simulink model "lateralControlTests"  (R2022a)
settings: Solver=VariableStepAuto  StartTime=0  StopTime=20  FixedStep=0.01  RelTol=1e-3
values from neighbouring files (symbols this model uses):
  Klat = place(A, B, poles)    [lat_sim_parameters.m]    (also in tuneLateralController.m)
  lr = 1.6    [acc_sim_parameters.m]    (also in lat_sim_parameters.m = 2; tuneLateralController.m = 2)
  m = 1575    [acc_sim_parameters.m]    (also in lat_sim_parameters.m = 2000; tuneLateralController.m = 2000)
  vx0 = 20    [lat_sim_parameters.m]    (also in tuneLateralController.m)
libraries: autolibshared x1
settings Model: Creator=Fernando VM  LastModifiedBy=fvall
settings SolverCC: AlgebraicLoopSolver=TrustRegion
settings DataIOCC: ExternalInput=[dt, da, dd]  ReturnWorkspaceOutputs=off
settings DebuggingCC: UnconnectedInputMsg=warning  UnconnectedOutputMsg=warning  UnconnectedLineMsg=warning  SFMachineParentedDataDiag=warning  ArithmeticOperatorsInVariantConditions=warning
settings SFSimCC: CustomCodeUndefinedFunction=UseInterfaceOnly

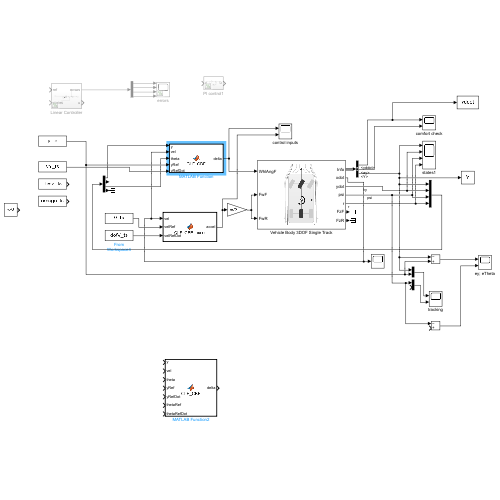
[thumbnail: Simulink's stored preview of the top-level diagram]
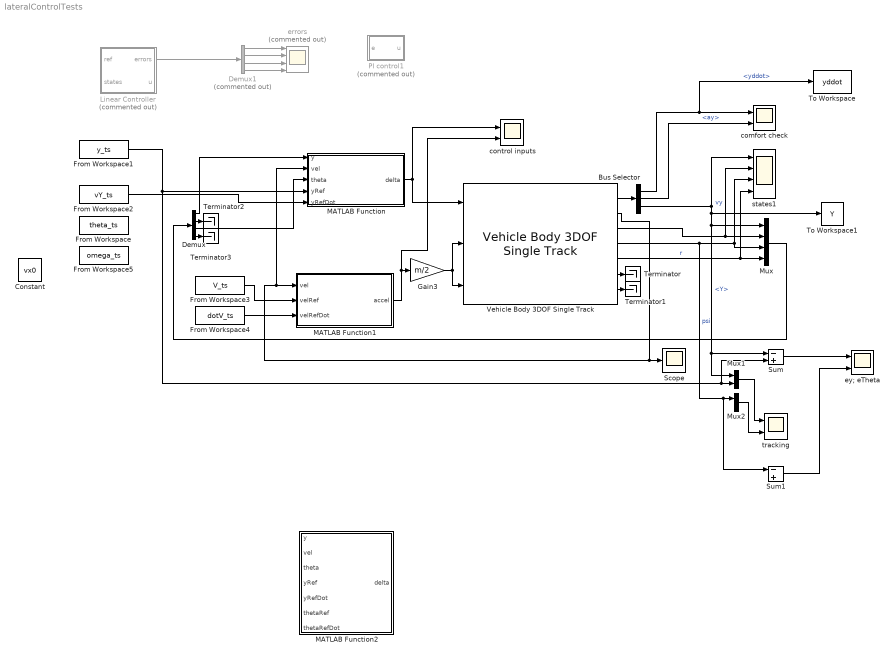
== system lateralControlTests ==
  Bus Selector : BusSelector  OutputSignals=BdyFrm.Cg.Acc.yddot,BdyFrm.Cg.Acc.ay,InertFrm.Cg.Disp.Y
  Constant : Constant  Value=vx0
  Demux : Demux
  Demux1 : Demux  Commented=on
  From Workspace : FromWorkspace  VariableName=theta_ts
  From Workspace1 : FromWorkspace  VariableName=y_ts
  From Workspace2 : FromWorkspace  VariableName=vY_ts
  From Workspace3 : FromWorkspace  VariableName=V_ts
  From Workspace4 : FromWorkspace  VariableName=dotV_ts
  From Workspace5 : FromWorkspace  VariableName=omega_ts
  Gain3 : Gain  Gain=m/2
  Linear Controller : Subsystem  Commented=on
  MATLAB Function : MATLAB Function  TreatAsAtomicUnit=on
  MATLAB Function1 : MATLAB Function  TreatAsAtomicUnit=on
  MATLAB Function2 : MATLAB Function  TreatAsAtomicUnit=on
  Mux : Mux
  Mux1 : Mux  Inputs=2
  Mux2 : Mux  Inputs=2
  PI control1 : Subsystem  Commented=on
  Scope : Scope
  Sum : Sum  Inputs=-+
  Sum1 : Sum  Inputs=-+
  Terminator{,1..3} (4 alike) : Terminator
  To Workspace : ToWorkspace  VariableName=yddot  SaveFormat=Timeseries  SampleTime=-1
  To Workspace1 : ToWorkspace  VariableName=Y  SaveFormat=Timeseries  SampleTime=-1
  Vehicle Body 3DOF Single Track : autolibshared/Vehicle Body 3DOF Single Track  trackMode=Single (bicycle)  inputMode=External longitudinal forces  frontSteerMode=on  rearSteerMode=off  windMode=off  muMode=off  extFMode=off  extMMode=off  htchFMode=off  htchMMode=off  extXo=off  extpsio=off  extxdoto=off  extro=off  extYo=off  extTamb=off  extydoto=off  aMode=2  NF=2  NR=2  m=m  a=lf  b=lr  h=0.35  dh=1  hh=0.2  X_o=0  xdot_o=vx0  CalphaMode=off  sigmaMode=on  d=0  hl=0  w=[1.4,1.4]  Cy_f=Cf  Cy_r=Cr  sigma_f=.1  sigma_r=.1  alpha_f_brk=[-.1 .1]  Cy_f_data=[-9e3 9e3]  alpha_r_brk=[-.1 .1]  Cy_r_data=[-9e3 9e3]  Y_o=0  ydot_o=0  Izz=Iz  psi_o=0  r_o=0  Af=2  Cd=.3  Cl=.1  Cpm=.1  beta_w=[0:0.01:0.3]  Cs=[0:0.03:0.9]  Cym=[0:0.01:0.3]  Pabs=101325  Tair=273  g=9.81  mu=1  xdot_tol=.01  Fznom=5000  Fxtire_sat=7e4  Fytire_sat=7e4  longOff=0  latOff=0  vertOff=0  wrapAng=off
      settings: SourceProductBaseCode=PW,DR,MT,VE
  comfort check : Scope  NumInputPorts=2
  control inputs : Scope  NumInputPorts=2
  errors : Scope  Commented=on  NumInputPorts=4
  ey; eTheta : Scope  NumInputPorts=2
  states1 : Scope  NumInputPorts=4
  tracking : Scope  NumInputPorts=2
  wires:
  Vehicle Body 3DOF Single Track/1 -> Bus Selector/1
  Bus Selector/3 -> To Workspace1/1, Sum/1, Mux1/1, Mux/1, states1/1  "<Y>"
  Vehicle Body 3DOF Single Track/3 -> states1/2, Mux/2  "vy"
  Vehicle Body 3DOF Single Track/4 -> Sum1/1, Mux2/1, Mux/3, states1/3  "psi"
  Gain3/1 -> Vehicle Body 3DOF Single Track/3, Vehicle Body 3DOF Single Track/2
  Vehicle Body 3DOF Single Track/2 -> MATLAB Function/2(vel), MATLAB Function1/1(vel), Scope/1
  Bus Selector/1 -> To Workspace/1, comfort check/1  "<yddot>"
  MATLAB Function1/1(accel) -> Gain3/1, control inputs/2
  Demux1/1 -> errors/1
  Demux1/2 -> errors/2
  Demux1/3 -> errors/3
  Demux1/4 -> errors/4
  Bus Selector/2 -> comfort check/2  "<ay>"
  Vehicle Body 3DOF Single Track/5 -> states1/4, Mux/4  "r"
  Vehicle Body 3DOF Single Track/6 -> Terminator/1
  Vehicle Body 3DOF Single Track/7 -> Terminator1/1
  Mux/1 -> Demux/1
  Linear Controller/1(errors) -> Demux1/1
  From Workspace1/1 -> MATLAB Function/4(yRef), Sum/2, Mux1/2
  MATLAB Function/1(delta) -> Vehicle Body 3DOF Single Track/1, control inputs/1
  Demux/1 -> MATLAB Function/1(y)
  Demux/2 -> Terminator2/1
  Demux/4 -> Terminator3/1
  From Workspace2/1 -> MATLAB Function/5(yRefDot)
  From Workspace3/1 -> MATLAB Function1/2(velRef)
  From Workspace4/1 -> MATLAB Function1/3(velRefDot)
  Mux1/1 -> tracking/1
  Mux2/1 -> tracking/2
  Sum/1 -> ey; eTheta/1
  Sum1/1 -> ey; eTheta/2
  Demux/3 -> MATLAB Function/3(theta)

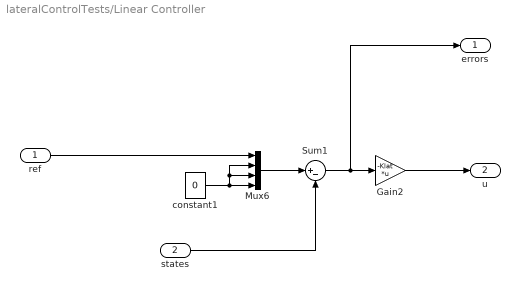
== system lateralControlTests/Linear Controller ==
  ref : Inport
  states : Inport  Port=2
  Gain2 : Gain  Gain=-Klat  Multiplication=Matrix(K*u)
  Mux6 : Mux
  Sum1 : Sum  Inputs=|+-
  constant1 : Constant  Value=0
  errors : Outport
  u : Outport  Port=2
  wires:
  constant1/1 -> Mux6/2, Mux6/3, Mux6/4
  states/1 -> Sum1/2
  Sum1/1 -> errors/1, Gain2/1
  Mux6/1 -> Sum1/1
  ref/1 -> Mux6/1
  Gain2/1 -> u/1

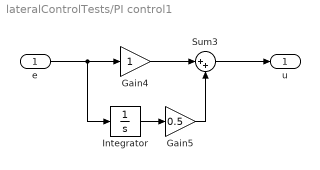
== system lateralControlTests/PI control1 ==
  e : Inport
  Gain4 : Gain
  Gain5 : Gain  Gain=0.5
  Integrator : Integrator
  Sum3 : Sum  Inputs=|++
  u : Outport  VectorParamsAs1DForOutWhenUnconnected=off
  wires:
  Gain5/1 -> Sum3/2
  Integrator/1 -> Gain5/1
  Gain4/1 -> Sum3/1
  Sum3/1 -> u/1
  e/1 -> Integrator/1, Gain4/1

== matlab function lateralControlTests/MATLAB Function1 ==
  data: vel input; velRef input; accel output; velRefDot input
function accel = CLF_CBF_accel(vel, velRef, velRefDot)

ev = velRef - vel;
psi0 = 2*ev*velRefDot + ev^2;
psi1 = -2*ev;
if psi0 > 0
    accel = -psi0/psi1;
else
    accel = 0;
end

== matlab function lateralControlTests/MATLAB Function ==
  data: y input; delta output; vel input; theta input; yRef input; yRefDot input
function delta = CLF_CBF(y, vel, theta, yRef, yRefDot)

wY=1;
wTheta=0;
lr = 2;

ey = yRef - y;
eTheta = -theta;
thetaRefDot = 0;

clf = wY*ey^2 + wTheta*eTheta^2;
kappaCLF = clf/2;
psi0 = 2*wY*ey*(yRefDot - vel*sin(theta)) + 2*wTheta*eTheta*thetaRefDot ...
    + kappaCLF;
psi1 = -2*wY*ey*vel*cos(theta) - 2*wTheta*eTheta*vel/lr;
if psi0 > 0
    betaCLF = -psi0/psi1;
else
    betaCLF = 0;
end

lr = 2;
lf = 3;
epsilon = 0.2;
% yDestLane = 4;
% barrierFunctionVal = yDestLane - y + epsilon;
% betaCBF = barrierFunctionVal / vel / cos(theta) - tan(theta);
% beta = min([betaCLF, betaCBF]);

k1 = 1/4;
lowerBoundCBF = (yRefDot - vel*sin(theta) + k1*(ey - epsilon)) ...
    / vel / cos(theta);
upperBoundCBF = (yRefDot - vel*sin(theta) + k1*(ey + epsilon)) ...
    / vel / cos(theta);

beta = min(max(betaCLF, lowerBoundCBF), upperBoundCBF);

delta = atan(tan(beta)*(lr+lf)/lr);

== matlab function lateralControlTests/MATLAB Function2 ==
  data: y input; delta output; vel input; theta input; yRef input; yRefDot input; thetaRef input; thetaRefDot input
function delta = CLF_CBF(y, vel, theta, yRef, yRefDot, thetaRef, thetaRefDot)

wY=1;
wTheta=1;
lr = 2;

ey = yRef - y;
eTheta = thetaRef-theta;

clf = wY*ey^2 + wTheta*eTheta^2;
kappaCLF = clf;
psi0 = 2*wY*ey*(yRefDot - vel*sin(theta)) + 2*wTheta*eTheta*thetaRefDot ...
    + kappaCLF;
psi1 = -2*wY*ey*vel*cos(theta) - 2*wTheta*eTheta*vel/lr;
if psi0 > 0
    betaCLF = -psi0/psi1;
else
    betaCLF = 0;
end

lr = 2;
lf = 3;
epsilon = 2;
yDestLane = 4;
barrierFunctionVal = yDestLane - y + epsilon;
betaCBF = barrierFunctionVal / vel / cos(theta) - tan(theta);
beta = min([betaCLF, betaCBF]);

% k1 = 1/4;
% lowerBoundCBF = (yRefDot - vel*sin(theta) + k1*(ey - epsilon)) ...
%     / vel / cos(theta);
% upperBoundCBF = (yRefDot - vel*sin(theta) + k1*(ey + epsilon)) ...
%     / vel / cos(theta);
% beta = min(max(betaCLF, lowerBoundCBF), upperBoundCBF);

delta = atan(tan(beta)*(lr+lf)/lr);
